simulink model "Integrated_model"  (R2017b)
settings: Solver=VariableStepAuto  StartTime=0.0  StopTime=10.0  RelTol=1e-3
model workspace (MAT data in the model file):
  H_Speed = 3600
  H_limit = 2500
  L_limit = 0
  inputVoltage = 5
  nBitConverter = 10
undefined symbols (not defined in the file): sigbuilder_block
libraries: simulink x2
(part 2 of 2)

== system Integrated_model/HVAC_System/HVAC_System/MotorSpeed_Calcn/temp_to_motorSpeed ==
  note: %age requirements
      |
      | input: AC temp value
      | output: motor speed value
      | logic: temp value is converted to motor value using two simple lookup tables covering from ( 16 - 32 deg C)
  note: Temperature_to_Motor_Speed_Conversion
  temp_input : Inport
  Temp_limiter : Saturate  UpperLimit=32  LowerLimit=25
      settings: AttributesFormatString=|
      | %<LowerLimit>
      | %<UpperLimit>
  Temp_limiter1 : Saturate  UpperLimit=26  LowerLimit=15
      settings: AttributesFormatString=|
      | %<LowerLimit>
      | %<UpperLimit>
  tempTomotor : Lookup_n-D  NumberOfTableDimensions=1  BreakpointsForDimension1=[25:32]  Table=[0 500 1000 1500 2000 2500 3000 3600]  InternalRulePriority=Speed  RndMeth=Simplest  InputSameDT=on
      settings: AttributesFormatString=%<RndMeth>
  tempTomotor1 : Lookup_n-D  NumberOfTableDimensions=1  BreakpointsForDimension1=[15:26]  Table=[0 3600 3400 3200 2800 2400 2000 1600 1300 900 500 0]  InternalRulePriority=Speed  RndMeth=Simplest  InputSameDT=on
      settings: AttributesFormatString=%<RndMeth>
  HeaterMotorSpeed : Outport
  CoolerMotorSpeed : Outport  Port=2
  wires:
  Temp_limiter1/1 -> tempTomotor1/1  "tempoutput"
  Temp_limiter/1 -> tempTomotor/1  "tempoutput"
  temp_input/1 -> Temp_limiter1/1, Temp_limiter/1  "temp_input"
  tempTomotor/1 -> HeaterMotorSpeed/1  "HeaterMotorSpeed"
  tempTomotor1/1 -> CoolerMotorSpeed/1  "CoolerMotorSpeed"

== system Integrated_model/Lighting_System/Automode/HeadLight_and_DayLight/FOr_comparing_with_daylight ==
  Out_High_beam_1 : Inport
  In_Light_Intensity : Inport  Port=2
  Compare_with_Daylight2 : RelationalOperator  OutDataTypeStr=boolean  RndMeth=Simplest
  Out_High_Beam : Outport
  wires:
  Out_High_beam_1/1 -> Compare_with_Daylight2/1  "Out_High_beam_1"
  Compare_with_Daylight2/1 -> Out_High_Beam/1  "Out_High_Beam"
  In_Light_Intensity/1 -> Compare_with_Daylight2/2  "In_Light_Intensity"

== system Integrated_model/Lighting_System/Automode/HeadLight_and_DayLight/For_COmparision_with_Daylight ==
  In_Intensity : Inport
  Out_Low_Beam_2 : Inport  Port=2
  Compare_with_Daylight : RelationalOperator  OutDataTypeStr=boolean  RndMeth=Simplest
  Out_Low_Beam : Outport
  wires:
  In_Intensity/1 -> Compare_with_Daylight/2  "In_Intensity"
  Out_Low_Beam_2/1 -> Compare_with_Daylight/1  "Out_Low_Beam_2"
  Compare_with_Daylight/1 -> Out_Low_Beam/1  "Out_Low_Beam"

== system Integrated_model/Lighting_System/Automode/HeadLight_and_DayLight/For_HeadLight ==
  In_Distance_sensor : Inport
  InStreet_Light : Inport  Port=2
  InReflection_opposite_vehicle : Inport  Port=3
  For_HeadLights : Stateflow chart  TreatAsAtomicUnit=on
  referrence_limit_value : Constant  Value=0.63
  Out_High_beam_1 : Outport
  Out_Low_Beam_2 : Outport  Port=2
  wires:
  InStreet_Light/1 -> For_HeadLights/2(InStreet_Light)  "InStreet_Light"
  In_Distance_sensor/1 -> For_HeadLights/1(In_Distance_sensor)  "In_Distance_sensor"
  InReflection_opposite_vehicle/1 -> For_HeadLights/3(InReflection_opposite_vehicle)  "InReflection_opposite_vehicle"
  referrence_limit_value/1 -> For_HeadLights/4(referrence_limit_value)  "referrence_limit_value"
  For_HeadLights/2(Out_Low_Beam_2) -> Out_Low_Beam_2/1  "Out_Low_Beam_2"
  For_HeadLights/1(Out_High_beam_1) -> Out_High_beam_1/1  "Out_High_beam_1"

== system Integrated_model/HVAC_System/HVAC_System/Automatic_Manual_system/Manual_Model/ManualSwitch ==
  note: %age Requirements
      |
      | input: voltage
      | input2: temperature
      | output: Final temp value
      | logic: Manual control for HVAC system
  note: Manual_Control_Subsystem
  autocontrol : Inport
  ManualInpts : Inport  Port=2
  Bitwise Operator : simulink/Logic and Bit Operations/Bitwise Operator  logicop=NOT  UseBitMask=off  BitMask=bin2dec('11011001')  BitMaskRealWorld=Stored Integer
  Product : Product
  Saturation : Saturate  UpperLimit=32  LowerLimit=16
      settings: AttributesFormatString=|
      | %<LowerLimit>
      | %<UpperLimit>
  ManualValue : Outport
  wires:
  Bitwise Operator/1 -> Product/1  "manualControl"
  ManualInpts/1 -> Saturation/1  "ManualInpts"
  Saturation/1 -> Product/2  "limitedop"
  autocontrol/1 -> Bitwise Operator/1  "autocontrol"
  Product/1 -> ManualValue/1  "ManualValue"

== stateflow chart Integrated_model/Wiper_system/WIPER_CONTROL_SYSTEM/Automatic_system/conditions ==
  (default) -> (junction 1) : {initial=0}
  (junction 1) -> (junction 5) [order 2] : [automatic>=40 & automatic<70]{Low=1,High=0,Medium=0}
  (junction 1) -> (junction 6) [order 3] : [automatic>=100 & automatic<=130]{High=1,Low=0,Medium=0}
  (junction 1) -> (junction 3) [order 1] : [automatic>=70 & automatic<100]{Medium=1,Low=0,High=0}
  (junction 5) -> (junction 22)
  (junction 6) -> (junction 22)
  (junction 3) -> (junction 22)
  data: automatic input; High output; Low output; Medium output; initial local

== stateflow chart Integrated_model/Window_control/Driver_control/driver ==
  state NormalState
    state Neutral
      entry:
      Up=0;
      Down=0;
    state Up
      entry:
      Up=1;
      Down=0;
    state Down
      entry:
      Up=0;
      Down=1;
    (default) -> Neutral
    Neutral -> Down [order 1] : [d_up==0&&d_down==1]
    Up -> Neutral [order 2] : [[d_up==0&&d_down==0]]
    Down -> Neutral [order 2] : [d_up==0&&d_down==0]
    Neutral -> Up [order 2] : [d_up==1&&d_down==0]
    Down -> Up [order 1] : [d_up==1&&d_down==0]
    Up -> Down [order 1] : [d_up==0&&d_down==1]
  state Obstacle
    entry:
    Up=0;
    Down=1;
  state Rain
    entry:
    Up=1;
    Down=0;
  (default) -> NormalState
  Rain -> Neutral : [Rain==0]
  Obstacle -> Neutral : [Obstacle==0]
  NormalState -> Obstacle [order 1] : [Obstacle==1]
  NormalState -> Rain [order 2] : [Rain==1]
  data: Obstacle input; Rain input; Up output; Down output; d_down input; d_up input

== stateflow chart Integrated_model/Central_lock_System/main_locking_system/voltagecombiner/to_lock_unlock ==
  note: LOGICTOLOCKANDUNLOCK
  note: %REQ:
      | here depending on the
      | value of finalvalue from adder
      | we get the status from this
      | chart depending on conditions
      | given.
      | input is 0 then status is 0
      | input is +ve then status 1
      | input is -ve then status -1
  (default) -> (junction 1)
  (junction 1) -> (junction 5) [order 2] : [finalvoltage>0]{status=1}
  (junction 1) -> (junction 8) [order 3] : [finalvoltage<0]{status=-1}
  (junction 1) -> (junction 3) [order 1] : [finalvoltage==0]{status=0}
  (junction 5) -> (junction 13)
  (junction 8) -> (junction 13)
  (junction 3) -> (junction 13)
  data: finalvoltage input; status output

== stateflow chart Integrated_model/Window_control/passenger_control/passenger ==
  state NormalState
    state Neutral
      entry:
      Up=0;
      Down=0;
    state Up
      entry:
      Up=1;
      Down=0;
    state Down
      entry:
      Up=0;
      Down=1;
    (default) -> Neutral
    Neutral -> Down [order 1] : [p_up==0&&p_down==1]
    Up -> Neutral [order 2] : [[p_up==0&&p_down==0]]
    Down -> Neutral [order 2] : [p_up==0&&p_down==0]
    Neutral -> Up [order 2] : [p_up==1&&p_down==0]
    Down -> Up [order 1] : [p_up==1&&p_down==0]
    Up -> Down [order 1] : [p_up==0&&p_down==1]
  state Obstacle
    entry:
    Up=0;
    Down=1;
  state Rain
    entry:
    Up=1;
    Down=0;
  (default) -> NormalState
  Rain -> Neutral : [Rain==0]
  Obstacle -> Neutral : [Obstacle==0]
  NormalState -> Obstacle [order 1] : [Obstacle==1]
  NormalState -> Rain [order 2] : [Rain==1]
  data: Obstacle input; Up output; Down output; Rain input; p_down input; p_up input

== stateflow chart Integrated_model/HVAC_System/HVAC_System/Automatic_Manual_system/Automatic_Model/Temp_sensor_to_Tvalue ==
  note: TempValue_Select_Model
  state Normal_temp
    en:
    DeH=0;
    state DehumifyingState
      en:
      DeH=1;
    state On_OffState
      en:
      DeH=0;
      Tvalue=0;
    (default) -> On_OffState
    On_OffState -> DehumifyingState : [DH>70]
    DehumifyingState -> On_OffState : [DH<70]
  state CoolerState
    en:
    DeH=0;
    Tvalue=25;
    state bet_23_24
      en:
      Tvalue=25;
    state bet_24_25
      en:
      Tvalue=24;
    state bet_25_27
      en:
      Tvalue=23;
    state bet_28_30
      en:
      Tvalue=21;
    state bet_27_28
      en:
      Tvalue=22;
    state bet_30_32
      en:
      Tvalue=20;
    state bet_32_33
      en:
      Tvalue=19;
    state bet_35_37
      en:
      Tvalue=17;
    state bet_33_35
      en:
      Tvalue=18;
    state grt_37
      en:
      Tvalue=16;
    (default) -> bet_23_24
    bet_24_25 -> bet_23_24 [order 2] : [T<25]
    bet_23_24 -> bet_24_25 : [T>24]
    bet_25_27 -> bet_24_25 [order 1] : [T<26]
    bet_24_25 -> bet_25_27 [order 1] : [T>25]
    bet_25_27 -> bet_27_28 [order 2] : [T>27]
    bet_27_28 -> bet_25_27 [order 2] : [T<28]
    bet_28_30 -> bet_27_28 [order 1] : [T<29]
    bet_27_28 -> bet_28_30 [order 1] : [T>28]
    bet_28_30 -> bet_30_32 [order 2] : [T>30]
    bet_30_32 -> bet_28_30 [order 2] : [T<31]
    bet_30_32 -> bet_32_33 [order 1] : [T>32]
    bet_32_33 -> bet_30_32 [order 1] : [T<33]
    bet_33_35 -> bet_32_33 [order 1] : [T<34]
    bet_32_33 -> bet_33_35 [order 2] : [T>33]
    bet_33_35 -> bet_35_37 [order 2] : [T>35]
    bet_35_37 -> bet_33_35 [order 2] : [T<36]
    grt_37 -> bet_35_37 : [T<38]
    bet_35_37 -> grt_37 [order 1] : [T>37]
  state HeaterState
    en:
    DeH=0;
    Tvalue=26;
    state at_20
      en:
      Tvalue=26;
    state bet_15_20
      en:
      Tvalue=27;
    state bet_10_15
      en:
      Tvalue=28;
    state bet_0_5
      en:
      Tvalue=30;
    state bet_5_10
      en:
      Tvalue=29;
    state bet_n5_0
      en:
      Tvalue=31;
    state less_n5
      en:
      Tvalue=32;
    (default) -> at_20
    bet_15_20 -> at_20 [order 2] : [T>19]
    at_20 -> bet_15_20 : [T<20]
    bet_10_15 -> bet_15_20 [order 1] : [T>14]
    bet_15_20 -> bet_10_15 [order 1] : [T<15]
    bet_10_15 -> bet_5_10 [order 2] : [T<10]
    bet_5_10 -> bet_10_15 [order 2] : [T>9]
    bet_0_5 -> bet_5_10 [order 1] : [T>4]
    bet_5_10 -> bet_0_5 [order 1] : [T<5]
    bet_0_5 -> bet_n5_0 [order 2] : [T<0]
    bet_n5_0 -> bet_0_5 [order 2] : [T>-1]
    bet_n5_0 -> less_n5 [order 1] : [T<-5]
    less_n5 -> bet_n5_0 : [T>-6]
  note: %age Requirements:
      |
      | input:Temperuture
      | input 2: humidity
      | output1:Temperature Value
      | output2: Dehumidifier Value
  (default) -> Normal_temp
  CoolerState -> On_OffState : [T<23]
  Normal_temp -> bet_23_24 [order 1] : [T>22]
  HeaterState -> On_OffState : [T>20]
  Normal_temp -> at_20 [order 2] : [T<21]
  data: Tvalue output; DeH output; T input; DH input

== stateflow chart Integrated_model/Lighting_System/Automode/HeadLight_and_DayLight/For_HeadLight/For_HeadLights ==
  state High_beam
    en:
    st=1;
    du:
    Out_High_beam_1=1;
    Out_Low_Beam_2=1;
  state Low_decrease
    en:
    st=2;
    du:
    Out_High_beam_1=0;
    Out_Low_Beam_2=In_Distance_sensor/25;
  state Low_turn_off
    en:
    st=4;
    du:
    Out_High_beam_1=0;
    Out_Low_Beam_2=0;
  state Low_beam
    en:
    st=3;
    du:
    Out_High_beam_1=0;
    Out_Low_Beam_2=1;
  note: % Requirements:
      | Inputs:
      | -> ux:Obstacle Distance sensing
      | ->uy: Reflection of the car opposite
      | ->uz: Street_Light_Detection
      | ->u_limit:Reflection light limit
      | Outputs:
      | ->u1:High Beam
      | ->u2:Low Beam
      | Logic:
      | ->When the obstacle is greater than 25 meters and Street_Light_Detection is less than 1 then the high beam,Low beam is turned ON
      | ->When the obstacle 5 to 25 meters the high beam is turned OFF and low beam is turned ON.Intensity depending on distance
      | ->When Obstacle is less than 5 meters and Street_Light_Detection is greater than 1 then Low beam Turned 'ON'
      | -> If Reflection light limit is more than the considered limit then turn off
      | low beam and if less turn on low beam
  High_beam -> Low_beam [order 2] : [In_Distance_sensor<=5 & InStreet_Light<1]
  High_beam -> Low_beam [order 3] : [InStreet_Light>=1]
  (default) -> High_beam
  Low_beam -> High_beam [order 2] : [In_Distance_sensor>50 & InStreet_Light<1]
  Low_decrease -> High_beam [order 2] : [In_Distance_sensor>25  & InStreet_Light<1]
  High_beam -> Low_decrease [order 1] : [In_Distance_sensor>5 &In_Distance_sensor<=25]
  Low_turn_off -> High_beam [order 3] : [In_Distance_sensor>25 & InStreet_Light<1]
  Low_beam -> Low_turn_off [order 3] : [InReflection_opposite_vehicle>referrence_limit_value &In_Distance_sensor<=5]
  Low_decrease -> Low_beam [order 3] : [In_Distance_sensor>5 & InStreet_Light>=1]
  Low_turn_off -> Low_beam [order 1] : [InReflection_opposite_vehicle<referrence_limit_value & In_Distance_sensor <=5]
  Low_beam -> Low_decrease [order 1] : [In_Distance_sensor>5&In_Distance_sensor<=25]
  Low_decrease -> Low_beam [order 1] : [In_Distance_sensor<=5]
  Low_turn_off -> Low_decrease [order 2] : [In_Distance_sensor>5 & In_Distance_sensor <=25]
  data: In_Distance_sensor input; Out_High_beam_1 output; Out_Low_Beam_2 output; InStreet_Light input; InReflection_opposite_vehicle input; referrence_limit_value input; st local

== stateflow chart Integrated_model/Lighting_System/Automode/Light_Indicator_/Day_light_intense ==
  state Sun_rise_set
    en:
    In_Light_Intensity=0.25;
  state night
    en:
    In_Light_Intensity=0.5;
  state Sunny
    en:
    In_Light_Intensity=0;
  state Dark_night
    en:
    In_Light_Intensity=1;
  note: %REQUIREMENTS:
      | Input:
      | ->f-Luminous intensity
      | Output:
      | ->Int-Intensity Maintainable
  (default) -> Sun_rise_set
  night -> Sun_rise_set : [f<1.5 && f>1]
  Sun_rise_set -> Sunny : [f>1.5]
  Sunny -> night [order 1] : [f>0.2 && f <1]
  Sunny -> Dark_night [order 2] : [f<0.2]
  Dark_night -> Sunny : [f>0.2]
  data: f input; In_Light_Intensity output
